simulink model "PMSM_FOC"  (R2024b)
settings: Solver=FixedStepDiscrete  StartTime=0.0  StopTime=5  FixedStep=0.0000002  RelTol=1e-3
libraries: slpidlib x2, simulink x2, spsDCVoltageSourceLib x1, spsPermanentMagnetSynchronousMachineLib x1, spsTwoLevelConverterLib x1, sps_lib x1
settings Model: Creator=14420  LastModifiedBy=14420

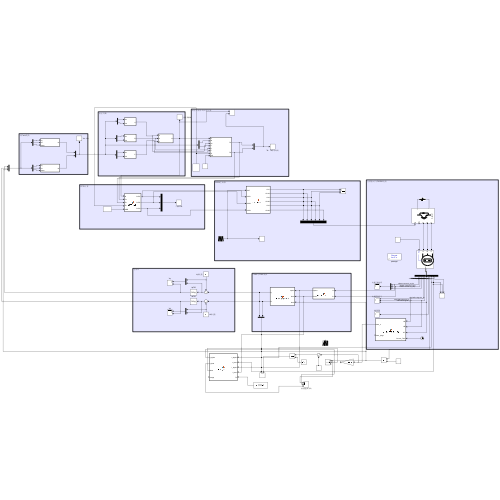
[thumbnail: Simulink's stored preview of the top-level diagram]
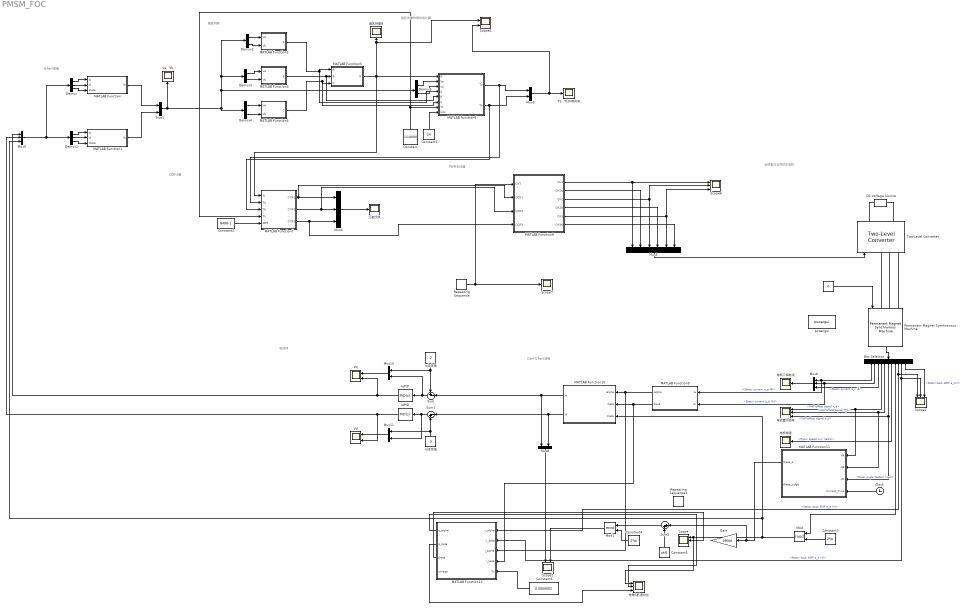
== system PMSM_FOC ==
  note: 电流环
  note: Clark与Park变换
  note: 全桥驱动与PMSM电机
  note: PWM生成器
  note: CCR计算
  note: 扇区矢量作用时间计算
  note: 扇区判断
  note: 反Park变换
  " " : Constant  Value=0
  Bus Selector : BusSelector  OutputSignals=Stator current is_a (A),Stator current is_b (A),Stator current is_c (A),Hall effect signal h_a,Hall effect signal h_b,Hall effect signal h_c,Rotor speed wm (rad/s),Rotor angle thetam (rad),Stator back EMF e_a (V),Stator back EMF e_b (V),Stator back EMF e_cV)
  Clock : Clock
  Constant : Constant  Value=1/10000
  Constant1 : Constant  Value=24
  Constant2 : Constant  Value=8400-1
  Constant3 : Constant  Value=2*pi
  Constant4 : Constant  Value=2*pi
  Constant5 : Constant  Value=pi/6
  Constant6 : Constant  Value=0.0000002
  DC Voltage Source : spsDCVoltageSourceLib/DC Voltage Source  Amplitude=24  Measurements=None
  Demux : Demux  Outputs=3
  Demux1 : Demux  Outputs=3
  Demux{2..5} (4 alike) : Demux  Outputs=2
  Gain : Gain  Gain=180/pi
  IdPID : slpidlib/PID Controller  Controller=PID  Form=Parallel  TimeDomain=Discrete-time  UseExternalTs=off  SampleTime=0.0001  IntegratorMethod=Forward Euler  FilterMethod=Forward Euler  ControllerParametersSource=internal  P=2  I=0  UseKiTs=off  D=0  UseExternalDerivativeSource=off  N=100  UseFilter=on  TunerSelectOption=Transfer Function Based (PID Tuner App)  InitialConditionSource=internal  InitialConditionForIntegrator=0  InitialConditionForFilter=0  DifferentiatorICPrevScaledInput=0  ExternalReset=none  TrackingMode=off  Kt=1  LimitOutput=off  SatLimitsSource=internal  UpperSaturationLimit=24  LowerSaturationLimit=-24  LinearizeAsGain=on  AntiWindupMode=none  Kb=1  LimitIntegrator=off  UpperIntegratorSaturationLimit=3  LowerIntegratorSaturationLimit=-3  POutMin=[]  POutMax=[]  IOutMin=[]  IOutMax=[]  DOutMin=[]  DOutMax=[]  NOutMin=[]  NOutMax=[]  SumOutMin=[]  SumOutMax=[]  SaturationOutMin=[]  SaturationOutMax=[]  PParamMin=[]  PParamMax=[]  IParamMin=[]  IParamMax=[]  DParamMin=[]  DParamMax=[]  NParamMin=[]  NParamMax=[]  KbParamMin=[]  KbParamMax=[]  KtParamMin=[]  KtParamMax=[]  KbOutMin=[]  KbOutMax=[]  KtOutMin=[]  KtOutMax=[]  IntegratorOutMin=[]  IntegratorOutMax=[]  FilterOutMin=[]  FilterOutMax=[]  SumI1OutMin=[]  SumI1OutMax=[]  SumI2OutMin=[]  SumI2OutMax=[]  SumI3OutMin=[]  SumI3OutMax=[]  SumI4OutMin=[]  SumI4OutMax=[]  SumDOutMin=[]  SumDOutMax=[]  DifferentiatorOutMin=[]  DifferentiatorOutMax=[]  FilterDiffOutCoefMin=[]  FilterDiffOutCoefMax=[]  ReciprocalOutMin=[]  ReciprocalOutMax=[]  SumDenOutMin=[]  SumDenOutMax=[]  SumNumOutMin=[]  SumNumOutMax=[]  DivideOutMin=[]  DivideOutMax=[]  UdiffTsProdOutMin=[]  UdiffTsProdOutMax=[]  NTsProdOutMin=[]  NTsProdOutMax=[]  UintegralTsProdOutMin=[]  UintegralTsProdOutMax=[]  UngainTsProdOutMin=[]  UngainTsProdOutMax=[]  ClampingZeroOutDataTypeStr=Inherit: Inherit via back propagation  ClampingZeroOutMin=[]  ClampingZeroOutMax=[]  FilterDenConstantOutDataTypeStr=Inherit: Inherit via back propagation  FilterDenConstantOutMin=[]  FilterDenConstantOutMax=[]  PCopyOutDataTypeStr=Inherit: Inherit via back propagation  PCopyOutMin=[]  PCopyOutMax=[]  NCopyOutDataTypeStr=Inherit: Inherit via back propagation  NCopyOutMin=[]  NCopyOutMax=[]  IntegratorContinuousStateAttributes=''  IntegratorStateMustResolveToSignalObject=off  IntegratorRTWStateStorageClass=Auto  FilterContinuousStateAttributes=''  FilterStateMustResolveToSignalObject=off  FilterRTWStateStorageClass=Auto  ParallelPVariant=InternalParameters  IdealPVariant=Disabled  IVariant=InternalParameters  DVariant=InternalParameters  IntegratorVariant=Discrete  SatVariant=Disabled  AWVariant=Passthrough  PCopyVariant=Disabled  TRVariant=Disabled  FdbkBlocksVariant=Forward  IdealPFdbkVariant=Disabled  SatFdbkVariant=Disabled  DerivativeFilterVariant=ForwardEulerFilter  NVariant=InternalParameters  NCopyVariant=Disabled  FilterICVariant=InternalICsFilter  IntegratorICVariant=InternalICs  ExternalResetVariant=Disabled  TRSumVariant=Passthrough  SumFdbkVariant=Disabled  SumVariant=Sum_PID  TsampFilterVariant=InternalTs  TsampNgainVariant=Passthrough  TsampIntegralVariant=Disabled_SignalSpec  ExternalSaturationOutDataTypeStr=Inherit: Same as second input  DerivativeSourceVariant=ErrorSignal  PreIntVariant=InternalPreInt
  IqPID : slpidlib/PID Controller  Controller=PID  Form=Parallel  TimeDomain=Discrete-time  UseExternalTs=off  SampleTime=0.0001  IntegratorMethod=Forward Euler  FilterMethod=Forward Euler  ControllerParametersSource=internal  P=2  I=0  UseKiTs=off  D=0  UseExternalDerivativeSource=off  N=100  UseFilter=on  TunerSelectOption=Transfer Function Based (PID Tuner App)  InitialConditionSource=internal  InitialConditionForIntegrator=0  InitialConditionForFilter=0  DifferentiatorICPrevScaledInput=0  ExternalReset=none  TrackingMode=off  Kt=1  LimitOutput=off  SatLimitsSource=internal  UpperSaturationLimit=24  LowerSaturationLimit=-24  LinearizeAsGain=on  AntiWindupMode=none  Kb=1  LimitIntegrator=off  UpperIntegratorSaturationLimit=3  LowerIntegratorSaturationLimit=-3  POutMin=[]  POutMax=[]  IOutMin=[]  IOutMax=[]  DOutMin=[]  DOutMax=[]  NOutMin=[]  NOutMax=[]  SumOutMin=[]  SumOutMax=[]  SaturationOutMin=[]  SaturationOutMax=[]  PParamMin=[]  PParamMax=[]  IParamMin=[]  IParamMax=[]  DParamMin=[]  DParamMax=[]  NParamMin=[]  NParamMax=[]  KbParamMin=[]  KbParamMax=[]  KtParamMin=[]  KtParamMax=[]  KbOutMin=[]  KbOutMax=[]  KtOutMin=[]  KtOutMax=[]  IntegratorOutMin=[]  IntegratorOutMax=[]  FilterOutMin=[]  FilterOutMax=[]  SumI1OutMin=[]  SumI1OutMax=[]  SumI2OutMin=[]  SumI2OutMax=[]  SumI3OutMin=[]  SumI3OutMax=[]  SumI4OutMin=[]  SumI4OutMax=[]  SumDOutMin=[]  SumDOutMax=[]  DifferentiatorOutMin=[]  DifferentiatorOutMax=[]  FilterDiffOutCoefMin=[]  FilterDiffOutCoefMax=[]  ReciprocalOutMin=[]  ReciprocalOutMax=[]  SumDenOutMin=[]  SumDenOutMax=[]  SumNumOutMin=[]  SumNumOutMax=[]  DivideOutMin=[]  DivideOutMax=[]  UdiffTsProdOutMin=[]  UdiffTsProdOutMax=[]  NTsProdOutMin=[]  NTsProdOutMax=[]  UintegralTsProdOutMin=[]  UintegralTsProdOutMax=[]  UngainTsProdOutMin=[]  UngainTsProdOutMax=[]  ClampingZeroOutDataTypeStr=Inherit: Inherit via back propagation  ClampingZeroOutMin=[]  ClampingZeroOutMax=[]  FilterDenConstantOutDataTypeStr=Inherit: Inherit via back propagation  FilterDenConstantOutMin=[]  FilterDenConstantOutMax=[]  PCopyOutDataTypeStr=Inherit: Inherit via back propagation  PCopyOutMin=[]  PCopyOutMax=[]  NCopyOutDataTypeStr=Inherit: Inherit via back propagation  NCopyOutMin=[]  NCopyOutMax=[]  IntegratorContinuousStateAttributes=''  IntegratorStateMustResolveToSignalObject=off  IntegratorRTWStateStorageClass=Auto  FilterContinuousStateAttributes=''  FilterStateMustResolveToSignalObject=off  FilterRTWStateStorageClass=Auto  ParallelPVariant=InternalParameters  IdealPVariant=Disabled  IVariant=InternalParameters  DVariant=InternalParameters  IntegratorVariant=Discrete  SatVariant=Disabled  AWVariant=Passthrough  PCopyVariant=Disabled  TRVariant=Disabled  FdbkBlocksVariant=Forward  IdealPFdbkVariant=Disabled  SatFdbkVariant=Disabled  DerivativeFilterVariant=ForwardEulerFilter  NVariant=InternalParameters  NCopyVariant=Disabled  FilterICVariant=InternalICsFilter  IntegratorICVariant=InternalICs  ExternalResetVariant=Disabled  TRSumVariant=Passthrough  SumFdbkVariant=Disabled  SumVariant=Sum_PID  TsampFilterVariant=InternalTs  TsampNgainVariant=Passthrough  TsampIntegralVariant=Disabled_SignalSpec  ExternalSaturationOutDataTypeStr=Inherit: Same as second input  DerivativeSourceVariant=ErrorSignal  PreIntVariant=InternalPreInt
  MATLAB Function : MATLAB Function  TreatAsAtomicUnit=on
  MATLAB Function1 : MATLAB Function  TreatAsAtomicUnit=on
  MATLAB Function10 : MATLAB Function  TreatAsAtomicUnit=on
  MATLAB Function11 : MATLAB Function  TreatAsAtomicUnit=on
  MATLAB Function12 : MATLAB Function  TreatAsAtomicUnit=on
  MATLAB Function2 : MATLAB Function  TreatAsAtomicUnit=on
  MATLAB Function3 : MATLAB Function  TreatAsAtomicUnit=on
  MATLAB Function4 : MATLAB Function  TreatAsAtomicUnit=on
  MATLAB Function5 : MATLAB Function  TreatAsAtomicUnit=on
  MATLAB Function6 : MATLAB Function  TreatAsAtomicUnit=on
  MATLAB Function7 : MATLAB Function  TreatAsAtomicUnit=on
  MATLAB Function8 : MATLAB Function  TreatAsAtomicUnit=on
  MATLAB Function9 : MATLAB Function  TreatAsAtomicUnit=on
  Mod : Math  Operator=mod
  Mod1 : Math  Operator=mod
  Mux{1,3,8,10..11} (5 alike) : Mux  Inputs=2
  Mux4 : Mux  Inputs=3
  Mux5 : Mux  Inputs=6
  Mux6 : Mux  Inputs=3
  Mux9 : Mux  Inputs=3
  Permanent Magnet Synchronous Machine : spsPermanentMagnetSynchronousMachineLib/Permanent Magnet Synchronous Machine  NbPhases=3  FluxDistribution=Trapezoidal  RotorType=Round  MechanicalLoad=Torque Tm  PresetModel=No  ShowDetailedParameters=on  MeasurementBus=off  Resistance=0.194  Inductance=0.000097  dqInductances=[8.5e-3,8.5e-3]  La=0.000835  MachineConstant=Torque Constant (N.m / A_peak)  Flux=0.015152  VoltageCst=22.2142  TorqueCst=0.21213  Flat=120  Mechanical=[0.000621417 0.000303448 7]  PolePairs=4  InitialConditions=[0,0, 0,0]  InitialConditions5ph=[0 0 0 0 0 0]  RefAngle=Aligned with phase A axis (original Park)  IterativeDiscreteModel=Trapezoidal non iterative  TsBlock=-1  TsPowergui=0
  Repeating Sequence : simulink/Sources/Repeating Sequence  rep_seq_t=[0 0.00005 0.0001]  rep_seq_y=[0 8400 0]
  Repeating Sequence1 : simulink/Sources/Repeating Sequence  rep_seq_t=[0 1]  rep_seq_y=[0 2*pi]
  Scope : Scope  NumInputPorts=3
  Scope1 : Scope  NumInputPorts=2
  Scope2 : Scope  NumInputPorts=3
  Scope4 : Scope  NumInputPorts=2
  Scope6 : Scope  NumInputPorts=3
  Scope7 : Scope
  Sum : Sum  Inputs=+-|
  Sum1 : Sum  Inputs=|-+
  Sum2 : Sum  Inputs=|++
  Ta、Tb作用时间 : Scope
  Two-Level Converter : spsTwoLevelConverterLib/Two-Level Converter  ModelType=Switching devices  Ron=1e-3  Rs=1e6  Cs=inf  Vforward=[0,0]  Ron_Diode=1e-3  Rs_Diode=1e6  Cs_Diode=inf  Vf_Diode=1e-3  Rs_CurrentSource=inf  Ron_ACsource=1e-3
      settings: LibrarySourceBlock=sps_lib/Power Electronics/Two-Level Converter
  Va、Vb : Scope
  Vd : Scope  NumInputPorts=2
  Vq : Scope  NumInputPorts=2
  id设定值 : Constant  Value=0
  iq设定值 : Constant  Value=2
  powergui : sps_lib/powergui  Priority=1  SimulationMode=Discrete  SampleTime=0.0000006  frequency=60  Iterations=50  frequencyindice=0  Pbase=100e6  ErrMax=1e-4  UnitsV=kV  UnitsW=MW  buscounter=0  FunctionMessages=off  echomessages=off  EnableUseOfTLC=off  CurrentSourceSwitches=off  DisableSnubberDevices=off  DisableRonSwitches=off  DisableVfSwitches=off  DisplayEquations=off  AutomaticDiscreteSolvers=off  SolverType=Tustin/Backward Euler (TBE)  Interpol=off  ExternalGateDelay=off  methode=off  Ts=100  x0status=blocks  SPID=on  SwTol=0  HookPort=off  NonlinearTolerance=1e-4  nMaxIteration=100  ContinueOnMaxIteration=off  RestoreLinks=warning  ResistiveCurrentMeasurement=off  Frange=[0:2:500]  Ylog=off  Xlog=on  ShowGrid=off  save=off  variable=ZData  structure=0  ZoomFFT=off  StartTime=0.0  cycles=1  DisplayStyle=1  fundamental=60  FreqAxis=off  MaxFrequency=1000  frequencyindicesteady=1  RmsSteady=1  display=off
  三相CCR : Scope
  扇区判据N : Scope
  电机三相电流 : Scope
  电机转速 : Scope
  电机霍尔信号 : Scope  NumInputPorts=3
  电角(速)度对比 : Scope  NumInputPorts=3
  wires:
  Mux1/1 -> Demux5/1, Demux3/1, Demux2/1, Demux4/1, Va、Vb/1
  MATLAB Function/1(Ia) -> Mux1/1
  MATLAB Function1/1(Ib) -> Mux1/2
  Demux1/2 -> MATLAB Function1/2(Id)
  Demux1/1 -> MATLAB Function1/1(Iq)
  Demux/2 -> MATLAB Function/2(Id)
  Demux/1 -> MATLAB Function/1(Iq)
  Demux1/3 -> MATLAB Function1/3(theta)
  Demux/3 -> MATLAB Function/3(theta)
  Demux2/1 -> MATLAB Function2/1(Va)
  Demux2/2 -> MATLAB Function2/2(Vb)
  Demux3/2 -> MATLAB Function3/2(Vb)
  Demux3/1 -> MATLAB Function3/1(Va)
  Demux4/1 -> MATLAB Function4/1(Va)
  Demux4/2 -> MATLAB Function4/2(Vb)
  MATLAB Function2/1(A) -> MATLAB Function6/4(A), MATLAB Function5/1(A)
  MATLAB Function4/1(C) -> MATLAB Function6/6(C), MATLAB Function5/3(C)
  MATLAB Function3/1(B) -> MATLAB Function6/5(B), MATLAB Function5/2(B)
  Demux5/1 -> MATLAB Function6/2(Va)
  Demux5/2 -> MATLAB Function6/3(Vb)
  Constant/1 -> MATLAB Function7/4(Tk), MATLAB Function6/7(Tk)
  Constant1/1 -> MATLAB Function6/8(Udc)
  Mux3/1 -> Scope4/2, Ta、Tb作用时间/1
  MATLAB Function6/1(Ta) -> MATLAB Function7/2(Ta), Mux3/1
  MATLAB Function6/2(Tb) -> MATLAB Function7/3(Tb), Mux3/2
  MATLAB Function7/1(CCR1) -> MATLAB Function8/2(CCR1), Mux4/1
  Mux4/1 -> 三相CCR/1
  MATLAB Function7/3(CCR3) -> MATLAB Function8/4(CCR3), Mux4/3
  MATLAB Function7/2(CCR2) -> MATLAB Function8/3(CCR2), Mux4/2
  MATLAB Function5/1(N) -> MATLAB Function7/1(N), MATLAB Function6/1(N), Scope4/1, 扇区判据N/1
  Constant2/1 -> MATLAB Function7/5(ARR)
  Repeating Sequence/1 -> Scope7/1, MATLAB Function8/1(CNT)
  MATLAB Function8/1(CH1) -> Mux5/1, Scope6/1
  MATLAB Function8/2(CH1N) -> Mux5/2
  MATLAB Function8/3(CH2) -> Mux5/3, Scope6/2
  MATLAB Function8/4(CH2N) -> Mux5/4
  MATLAB Function8/5(CH3) -> Scope6/3, Mux5/5
  MATLAB Function8/6(CH3N) -> Mux5/6
  Mux5/1 -> Two-Level Converter/1
  " "/1 -> Permanent Magnet Synchronous Machine/1
  Permanent Magnet Synchronous Machine/1 -> Bus Selector/1
  Mux6/1 -> 电机三相电流/1
  Bus Selector/1 -> MATLAB Function9/1(ia), Mux6/1  "<Stator current is_a (A)>"
  Bus Selector/2 -> MATLAB Function9/2(ib), Mux6/2  "<Stator current is_b (A)>"
  Bus Selector/3 -> Mux6/3  "<Stator current is_c (A)>"
  Bus Selector/4 -> 电机霍尔信号/1, MATLAB Function11/1(HA)  "<Hall effect signal h_a>"
  Bus Selector/5 -> 电机霍尔信号/2, MATLAB Function11/2(HB)  "<Hall effect signal h_b>"
  Bus Selector/6 -> 电机霍尔信号/3, MATLAB Function11/3(HC)  "<Hall effect signal h_c>"
  Bus Selector/7 -> 电机转速/1  "<Rotor speed wm (rad/s)>"
  MATLAB Function9/1(ialpha) -> MATLAB Function12/3(i_alpha), MATLAB Function10/1(ialpha)
  MATLAB Function9/2(ibeta) -> MATLAB Function12/4(i_beta), MATLAB Function10/2(ibeta)
  MATLAB Function10/2(id) -> Sum1/1, Mux8/2
  Mux8/1 -> Scope1/1
  Sum/1 -> Mux10/2, IqPID/1
  iq设定值/1 -> Sum/1, Mux10/1
  MATLAB Function10/1(iq) -> Mux8/1, Sum/2
  Sum1/1 -> Mux11/2, IdPID/1
  id设定值/1 -> Mux11/1, Sum1/2
  IqPID/1 -> Vq/2, Mux9/1
  IdPID/1 -> Vd/2, Mux9/2
  Mux9/1 -> Demux/1, Demux1/1
  Mux10/1 -> Vq/1
  Mux11/1 -> Vd/1
  Bus Selector/8 -> Mod/1  "<Rotor angle thetam (rad)>"
  MATLAB Function11/1(theta_e) -> Sum2/1, Gain/1
  Mod/1 -> Mux9/3, MATLAB Function10/3(theta), 电角(速)度对比/1, Scope/1
  Constant3/1 -> Mod/2
  Clock/1 -> MATLAB Function11/4(Current_Time)
  Sum2/1 -> Mod1/1
  Constant4/1 -> Mod1/2
  Mod1/1 -> Scope1/2
  Constant5/1 -> Sum2/2
  Constant6/1 -> MATLAB Function12/5(Ts)
  MATLAB Function12/1(e_alpha) -> 电角(速)度对比/2
  Bus Selector/9 -> Scope2/1, MATLAB Function12/1(v_alpha)  "<Stator back EMF e_a (V)>"
  Bus Selector/10 -> Scope2/2, MATLAB Function12/2(v_beta)  "<Stator back EMF e_b (V)>"
  Bus Selector/11 -> Scope2/3  "<Stator back EMF e_cV)>"
  MATLAB Function12/2(e_beta) -> 电角(速)度对比/3
  MATLAB Function12/3(theta) -> Scope/2
  connections:
  Permanent Magnet Synchronous Machine/LConn1 -- Two-Level Converter/LConn1
  Permanent Magnet Synchronous Machine/LConn2 -- Two-Level Converter/LConn2
  Permanent Magnet Synchronous Machine/LConn3 -- Two-Level Converter/LConn3
  DC Voltage Source/RConn1 -- Two-Level Converter/RConn1
  DC Voltage Source/LConn1 -- Two-Level Converter/RConn2

== matlab function PMSM_FOC/MATLAB Function9 ==
  data: ia input; ialpha output; ib input; ibeta output
function [ialpha,ibeta] = ClarkTransformer(ia,ib)
ialpha = ia;
ibeta = (ia + 2*ib) / sqrt(3);
end

== matlab function PMSM_FOC/MATLAB Function10 ==
  data: ialpha input; iq output; ibeta input; id output; theta input
function [iq,id] = ParkTransformer(ialpha,ibeta,theta)
id = ialpha*cos(theta) + ibeta*sin(theta);
iq = -ialpha*sin(theta) + ibeta*cos(theta);
end

== matlab function PMSM_FOC/MATLAB Function11 ==
  data: HA input; theta_e output; HB input; HC input; Current_Time input; theta_judge output
function [theta_e, theta_judge] = Hall_To_FOC_Fix_180(HA, HB, HC, Current_Time)
% 霍尔传感器连续电角度计算（带时间线性插值）
% 输入：HA,HB,HC (0/1)，Current_Time 当前仿真时间（标量，s）
% 输出：theta_e   —— 连续电角度（rad，无符号，随时间线性增加）
%       theta_judge —— 当前扇区离散角度（rad，用于检测）

    persistent init_flag
    persistent last_time         % 上次霍尔状态变化时的仿真时间
    persistent last_angle        % 上次变化时的连续角度
    persistent prev_judge        % 上次扇区角度（用于检测变化）
    persistent omega_est         % 估算的电角速度 (rad/s)

    % ---------- 初始化 ----------
    if isempty(init_flag)
        last_time   = Current_Time;
        last_angle  = 0;
        prev_judge  = -1;          % 初始为无效值
        omega_est   = 0;
        init_flag   = true;
    end

    % ---------- 根据霍尔编码查表得到当前扇区角度 ----------
    code = HA*4 + HB*2 + HC;
    switch code
        case 1
            theta_judge = 4*pi/3;
        case 2
            theta_judge = 2*pi/3;
        case 3
            theta_judge = pi;
        case 4
            theta_judge = 0;
        case 5
            theta_judge = 5*pi/3;
        case 6
            theta_judge = pi/3;
        otherwise
            theta_judge = prev_judge;   % 无效状态保持上一次
    end

    % ---------- 检测霍尔状态是否变化 ----------
    % 注意：首次检测到有效状态时，只记录时间，不做速度估算
    if theta_judge ~= prev_judge && prev_judge ~= -1
        % 计算本次变化的角增量（处理 -2π 到 +2π 的环绕）
        delta_angle = theta_judge - prev_judge;
        delta_angle = mod(delta_angle + pi, 2*pi) - pi;   % 归一化到 [-pi, pi]

        % 计算两次变化之间的时间间隔
        dt_event = Current_Time - last_time;
        if dt_event > 1e-12
            % 估算当前平均速度
            omega_est = delta_angle / dt_event;
        end

        % 更新基准角度（实际连续角度累加）
        last_angle = last_angle + delta_angle;
        % 更新时间基准
        last_time = Current_Time;
    end

    % 如果是第一次有效状态，设定初始基准
    if prev_judge == -1 && theta_judge ~= -1
        last_time  = Current_Time;
        last_angle = theta_judge;     % 从当前扇区角度开始
        omega_est  = 0;               % 初始速度未知，设为0
    end

    % 更新上一次扇区角度（用于下次判断）
    prev_judge = theta_judge;

    % ---------- 在当前扇区内根据时间线性外推 ----------
    dt = Current_Time - last_time;
    theta_ea = last_angle + omega_est * dt - pi/3;
    theta_e = mod(theta_ea, 2*pi);

    % 注意：theta_e 可能会因速度估算误差而略有漂移，但每个霍尔事件会修正一次。
end

== matlab function PMSM_FOC/MATLAB Function12 ==
  data: v_alpha input; e_alpha output; v_beta input; i_alpha input; i_beta input; Ts input; e_beta output; theta output; omega output
function [e_alpha, e_beta, theta, omega] = SMO_noPLL(v_alpha, v_beta, i_alpha, i_beta, Ts)
%#codegen

% ---------- 电机参数 ----------
L = 0.097e-3;       % 相电感 (H)
R = 0.194;          % 相电阻 (Ohm)
k = 40;             % 滑模增益，需 > max(|反电动势|)
fc = 200;           % 反电动势低通滤波截止频率 (Hz)
fc_omega = 50;      % 速度低通滤波截止频率 (Hz)，用于平滑速度估算
E_min = 0.5;        % 反电动势幅值死区 (V)，低于此值时保持上一角度

% ---------- 持久变量 ----------
persistent i_alpha_hat i_beta_hat e_alpha_f e_beta_f
persistent theta_last omega_f

if isempty(i_alpha_hat)
    i_alpha_hat = 0;
    i_beta_hat = 0;
    e_alpha_f  = 0;
    e_beta_f   = 0;
    theta_last = 0;
    omega_f    = 0;
end

% ---------- 1. 滑模控制律 ----------
error_alpha = i_alpha_hat - i_alpha;
error_beta  = i_beta_hat  - i_beta;

z_alpha = k * sign(error_alpha);
z_beta  = k * sign(error_beta);

% ---------- 2. 电流观测器动态 ----------
di_alpha = (v_alpha - R * i_alpha_hat - z_alpha) / L;
di_beta  = (v_beta  - R * i_beta_hat  - z_beta ) / L;

i_alpha_hat = i_alpha_hat + Ts * di_alpha;
i_beta_hat  = i_beta_hat  + Ts * di_beta;

% ---------- 3. 等效控制量低通滤波 → 反电动势 ----------
alpha_lpf = 1 - exp(-2 * pi * fc * Ts);
e_alpha_f = (1 - alpha_lpf) * e_alpha_f + alpha_lpf * z_alpha;
e_beta_f  = (1 - alpha_lpf) * e_beta_f  + alpha_lpf * z_beta;

e_alpha = e_alpha_f;
e_beta  = e_beta_f;

% ---------- 4. 直接角度计算（去掉了PLL）----------
E = sqrt(e_alpha_f^2 + e_beta_f^2);
if E > E_min
    % 反电动势与电角度关系: e_alpha = -E*sinθ, e_beta = E*cosθ
    theta_raw = atan2(-e_alpha_f, e_beta_f);
    % 解算速度（后向差分，单位 rad/s）
    omega_raw = (theta_raw - theta_last) / Ts;
    theta_last = theta_raw;
else
    % 反电动势太弱，保持上一时刻角度，速度置零（或维持）
    theta_raw = theta_last;
    omega_raw = 0;
end

% 角度归一化到 [0, 2π)
theta = mod(theta_raw, 2*pi);

% 速度低通滤波，减少差分噪声
alpha_omega = 1 - exp(-2 * pi * fc_omega * Ts);
omega_f = (1 - alpha_omega) * omega_f + alpha_omega * omega_raw;
omega = omega_f;

end

== matlab function PMSM_FOC/MATLAB Function1 ==
  data: Iq input; Id input; Ib output; theta input
function Ib = Calculate_Ib(Iq,Id,theta)
Ib = Id*sin(theta) + Iq*cos(theta);
end

== matlab function PMSM_FOC/MATLAB Function ==
  data: Iq input; Id input; Ia output; theta input
function Ia = Calculate_Ia(Iq,Id,theta)
Ia = Id*cos(theta) - Iq*sin(theta);
end

== matlab function PMSM_FOC/MATLAB Function2 ==
  data: Va input; Vb input; A output
function A = fcn(Va,Vb)
A = Vb;
end

== matlab function PMSM_FOC/MATLAB Function3 ==
  data: Va input; Vb input; B output
function B = fcn(Va,Vb)
B = sqrt(3)*Va/2 - Vb/2;
end

== matlab function PMSM_FOC/MATLAB Function4 ==
  data: Va input; Vb input; C output
function C = fcn(Va,Vb)
C = -sqrt(3)*Va/2 - Vb/2;
end

== matlab function PMSM_FOC/MATLAB Function5 ==
  data: A input; B input; C input; N output
function N = SectorJudge(A, B, C)
N = 0;
if(A > 0)
    N = N + 1;
end
if(B > 0)
    N = N + 2;
end
if(C > 0)
    N = N + 4;
end
end

== matlab function PMSM_FOC/MATLAB Function6 ==
  data: N input; Va input; Ta output; Vb input; A input; B input; C input; Tk input; Udc input; Tb output
function [Ta,Tb] = VectorTimeCalculate(N,Va,Vb,A,B,C,Tk,Udc)

Ta = double(0);
Tb = double(0);

X = sqrt(3)*Tk/Udc;

if(N == 1)
   Ta = X * -B;
   Tb = X * -C;
end
if(N == 2)
   Ta = X * -C;
   Tb = X * -A;
end
if(N == 3)
   Ta = X * B;
   Tb = X * A;
end
if(N == 4)
   Ta = X * -A;
   Tb = X * -B;
end
if(N == 5)
   Ta = X * A;
   Tb = X * C;
end
if(N == 6)
   Ta = X * C;
   Tb = X * B;
end
if (Ta + Tb) > Tk
    % 等比例缩小（保持电压矢量角度不变，只压缩幅值）
    Ta = Ta / (Ta + Tb) * Tk;
    Tb = Tb / (Ta + Tb) * Tk;
end
end

== matlab function PMSM_FOC/MATLAB Function7 ==
  data: N input; CCR1 output; CCR2 output; CCR3 output; Ta input; Tb input; Tk input; ARR input
function [CCR1,CCR2,CCR3] = CCRCalculate(N,Ta,Tb,Tk,ARR)
CCR1 = double(0);
CCR2 = double(0);
CCR3 = double(0);
value1 = (Tk-Ta-Tb)*ARR*10000/4.0;
value2 = value1 + Ta*ARR*10000/2.0;
value3 = value2 + Tb*ARR*10000/2.0;

switch(N)
    case 3
        CCR1 = value1;
        CCR2 = value2;
        CCR3 = value3;
    case 1
        CCR1 = value2;
        CCR2 = value1;
        CCR3 = value3;
    case 5
        CCR1 = value3;
        CCR2 = value1;
        CCR3 = value2;
    case 4
        CCR1 = value3;
        CCR2 = value2;
        CCR3 = value1;
    case 6
        CCR1 = value2;
        CCR2 = value3;
        CCR3 = value1;
    case 2
        CCR1 = value1;
        CCR2 = value3;
        CCR3 = value2;
end

== matlab function PMSM_FOC/MATLAB Function8 ==
  data: CNT input; CH1 output; CCR1 input; CCR2 input; CCR3 input; CH1N output; CH2 output; CH2N output; CH3 output; CH3N output
function [CH1,CH1N,CH2,CH2N,CH3,CH3N] = PWMGenerator(CNT,CCR1,CCR2,CCR3)

CH1 = 0;
CH1N = 0;
CH2 = 0;
CH2N = 0;
CH3 = 0;
CH3N = 0;

if(CNT>CCR1)
    CH1 = 1;
    CH1N = 0;
else
    CH1 = 0;
    CH1N = 1;
end
if(CNT>CCR2)
    CH2 = 1;
    CH2N = 0;
else
    CH2 = 0;
    CH2N = 1;
end
if(CNT>CCR3)
    CH3 = 1;
    CH3N = 0;
else
    CH3 = 0;
    CH3N = 1;
end
end
